simulink library "AnnVolumeBtc"  (R2022b)
settings: Solver=VariableStepAuto  StartTime=0.0  StopTime=10.0  RelTol=1e-3
undefined symbols (not defined in the file or in its folder): Row
libraries: TuneVar x4, TOP x2, FeaturePath x1, HandyTextFile x1, RTC x1, RgainyBtc x1
settings Model: Creator=yp1048186  LastModifiedBy=kl13806
settings SolverCC: AlgebraicLoopSolver=TrustRegion
settings DebuggingCC: UnconnectedInputMsg=warning  UnconnectedOutputMsg=warning  UnconnectedLineMsg=warning  SFMachineParentedDataDiag=warning
settings ModelReferenceCC: EnableRefExpFcnMdlSchedulingChecks=on
settings RTWCC: DLArmComputeVersion=19.05

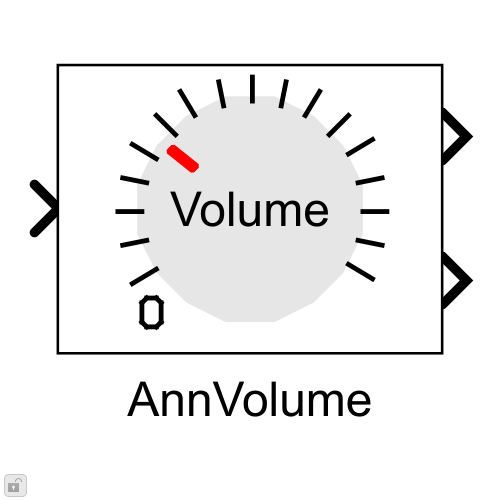
[thumbnail: Simulink's stored preview of the top-level diagram]
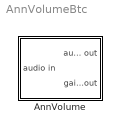
== system AnnVolumeBtc ==
  AnnVolume : Subsystem  mask(Blocklib AnnVolume){FeatureName=Volume, Config=[], TriggerInit=[815 415 895 475]}
      mask prompts: FeatureName "Feature path name:"; Config "AnnVolumeConfig"; TriggerInit "Hidden: MoveFcn redraw"
      mask help: This volume signal block includes receipt of volume level (via RTC) as well as tuning variables to calibrate a gain table that maps 8-bit integer volume index (from RTC) to float decibels.
      mask init:
      | blkh=gcbh;
      | Config=BTConfig.Assert(blkh,Config);
      | BTConfig.InitSetFeatureIfPresent(blkh,'FeatureName');
      | Config.Validate();
      settings: MoveFcn=VolumeMask.CB_TriggerInit(gcbh);
      mask TypeOptions FeatureName: FeaturePath/FeatureName
      mask Callback Config: BTConfig.CallbackHideIfPresent(gcbh,{'FeatureName'});
      mask Callback TriggerInit: VolumeMask.CB_TriggerInit(gcbh);
      mask Display:
      | [path,w,h] = IconVolumeMask();
      | 
      | % work in pixels since the icon does not scale
      | pos = get(gcbh,'position');
      | bw = pos(3) - pos(1);
      | bh = pos(4) - pos(2);
      | 
      | % Draw centered icon
      | xAdj = bw/2 - w/2;
      | yAdj = bh/2 - h/2;
      | for i=1:length(path)
      |     if (path(i).rgb(1) >= 0)
      |         patch(path(i).x+xAdj, path(i).y+yAdj, path(i).rgb);
      |     end
      |     if (path(i).stroke(1) >= 0)
      |         plot(path(i).x+xAdj, path(i).y+yAdj);
      |     end
      | end
      | 
      | % Display some text
      | text(bw/2, bh/2,FeatureName, ...
      |     'horizontalAlignment','center', ...
      |     'VerticalAlignment','middle');

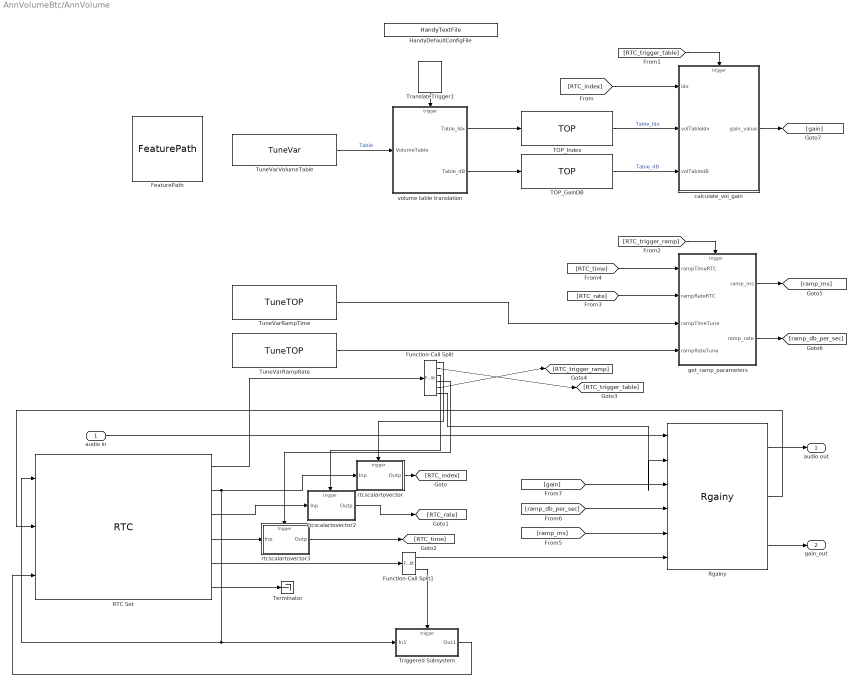
== system AnnVolumeBtc/AnnVolume ==
  audio in : Inport
  FeaturePath : FeaturePath/FeaturePath  FeatureName=Volume  IsGroup=off  GroupNumber=-1  IsModule=off  TriggerInit=[-260 -306 -145 -199]
      settings: SourceProductName=Bose Talaria
  Function-Call Split : FunctionCallSplit  IconShape=distinctive  NumOutputPorts=6
  Function-Call Split1 : FunctionCallSplit  IconShape=distinctive  NumOutputPorts=2  OutputPortLayout=default
  HandyDefaultConfigFile : HandyTextFile/HandyTextFile  TemplateSource=Config  FileSuffix=Init  OpenDialogOnLoad=off  UseThisBlockName=off  TheDefaultText=|  ShowInLibBrowser=on
      | % $(FILENAME) Setup model parameters for each "Init" callback (e.g. update diagram)
      | sample_rate_in_hertz = 44100;
      | frame_size = 32;
      | sysin_channel_count = 2;
      settings: SourceProductName=Bose Talaria
  RTC Set : RTC/RTC  Description=|  REQ_Priority=RTC_Mask.NormalPriority  RequestAtInit=off  EnableRequest=on  REQElemName1=volume_index  REQElemType1=uint32  REQElemWidth1=Config.NumInputChannels  REQElemInitial1=[]  REQElemName2=db_per_second  REQElemType2=uint32  REQElemWidth2=Config.NumInputChannels  REQElemInitial2=[]  REQElemName3=ramp_milliseconds  REQElemType3=uint32  REQElemWidth3=Config.NumInputChannels  REQElemInitial3=[]  REQElemType4=uint32  REQElemWidth4=1  REQElemInitial4=[]  REQElemType5=uint32  REQElemWidth5=1  REQElemInitial5=[]  REQElemType6=uint32  REQElemWidth6=1  REQElemInitial6=[]  REQElemType7=uint32  REQElemWidth7=1  REQElemInitial7=[]  REQElemType8=uint32  REQElemWidth8=1  REQElemInitial8=[]  REQElemType9=uint32  REQElemWidth9=1  REQElemInitial9=[]  REQElemType10=uint32  REQElemWidth10=1  REQElemInitial10=[]  EnableResponse=on  EnableRSP_StatusIn=off  RSPElemName1=gain_index  RSPElemType1=uint32  RSPElemWidth1=Config.NumInputChannels  RSPElemType2=uint32  RSPElemWidth2=1  RSPElemType3=uint32  RSPElemWidth3=1  RSPElemType4=uint32  RSPElemWidth4=1  RSPElemType5=uint32  RSPElemWidth5=1  RSPElemType6=uint32  RSPElemWidth6=1  RSPElemType7=uint32  RSPElemWidth7=1  RSPElemType8=uint32  RSPElemWidth8=1  RSPElemType9=uint32  RSPElemWidth9=1  RSPElemType10=uint32  RSPElemWidth10=1  EnableNotification=on  EnableNTF_PrepTrig=on  NTFElemName1=gain_index  NTFElemType1=uint32  NTFElemWidth1=Config.NumInputChannels  NTFElemType2=uint32  NTFElemWidth2=1  NTFElemType3=uint32  NTFElemWidth3=1  NTFElemType4=uint32  NTFElemWidth4=1  NTFElemType5=uint32  NTFElemWidth5=1  NTFElemType6=uint32  NTFElemWidth6=1  NTFElemType7=uint32  NTFElemWidth7=1  NTFElemType8=uint32  NTFElemWidth8=1  NTFElemType9=uint32  NTFElemWidth9=1  NTFElemType10=uint32  NTFElemWidth10=1  MaskMessageName=Set
      | Sets new target volume.
      | Provide the target volume as 8 bit index value to be mapped through a tunable VolumeTable.
      |  
      | To use slope-based ramping:
      | ----------------------------------
      | When db_per_second has a non-zero value,ramp_milliseconds is ignored and db_per_second controls the ramp.
      |  
      | To use time-based ramping:
      | ----------------------------------
      | The value of db_per_second must be zero for ramp milliseconds to then control the ramping.
      settings: SourceProductName=Bose Talaria
  Rgainy : RgainyBtc/Rgainy  GainOutEnable=on  Config=Config.Rgainy
  TOP_GainDB : TOP/TOP  TriggerInit=[380 -243 530 -187]  TopName=Table_dB  DataType=Inherit: Same as input  BankNumber=Config.BankNumber  PreOverlay=false  PostOverlay=false  Role=Automatic
      settings: SourceProductName=Bose Talaria
  TOP_Index : TOP/TOP  TriggerInit=[380 -313 530 -257]  TopName=Table_Idx  DataType=Inherit: Same as input  BankNumber=Config.BankNumber  PreOverlay=false  PostOverlay=false  Role=Automatic
      settings: SourceProductName=Bose Talaria
  Terminator : Terminator
  TranslateTrigger1 : TuneVar/TranslateTrigger  TriggerInit=[211 -395 249 -345]
      settings: SourceProductName=Bose Talaria
  Triggered Subsystem : Subsystem  TreatAsAtomicUnit=on
  TuneVarRampRate : TuneVar/TuneTOP  TriggerInit=[-95 52 75 108]  TopName=RampRate  TuneName=RampRate  DataType=single  TunabilityNumber=2  MinValue=5  MaxValue=50000  BankNumber=0  PreOverlay=false  PostOverlay=false  UseSameName=on  MaskValue=100
      settings: SourceProductName=Bose Talaria
  TuneVarRampTime : TuneVar/TuneTOP  TriggerInit=[-95 -28 75 28]  TopName=RampTime  TuneName=RampTime  DataType=single  TunabilityNumber=1  MinValue=[]  MaxValue=[]  BankNumber=0  PreOverlay=false  PostOverlay=false  UseSameName=on  MaskValue=100
      settings: SourceProductName=Bose Talaria
  TuneVarVolumeTable : TuneVar/TuneVar  Description=|  TuneName=Table  SpecifyMaxSize=on  VariableDim=1 (Row)  MaxSize=[16 2]  TunabilityNumber=2  MinValue=[0;-100]  MaxValue=[1;0]  TriggerInit=[-95 -275 75 -225]  MaskValue=[[1 32 64 96 128 160 192 224] / 255; [-126.5 -100 -90 -40 -30 -20 -10 0.0]]'
      | <HTML>Gain table maps index to gain.
      | The index values are <FONT color="red">normalized</Font> floats between 0 and 1 while the gains are in dB (i.e. 0 implies no attenuation).
      | </html>
      settings: SourceProductName=Bose Talaria
  calculate_vol_gain : MATLAB Function  TreatAsAtomicUnit=on
  get_ramp_parameters : MATLAB Function  TreatAsAtomicUnit=on
  rtcscalartovector : MATLAB Function  TreatAsAtomicUnit=on
  rtcscalartovector2 : MATLAB Function  TreatAsAtomicUnit=on
  rtcscalartovector3 : MATLAB Function  TreatAsAtomicUnit=on
  volume table translation : MATLAB Function  TreatAsAtomicUnit=on
  audio out : Outport  VectorParamsAs1DForOutWhenUnconnected=off
  gain_out : Outport  Port=2  VectorParamsAs1DForOutWhenUnconnected=off
  wires:
  Rgainy/1 -> audio out/1
  volume table translation/2(Table_dB) -> TOP_GainDB/1
  volume table translation/1(Table_Idx) -> TOP_Index/1
  TuneVarVolumeTable/1 -> volume table translation/1(VolumeTable)  "Table"
  TranslateTrigger1/1 -> volume table translation/Trigger
  TOP_Index/1 -> calculate_vol_gain/2(volTableIdx)  "Table_Idx"
  TOP_GainDB/1 -> calculate_vol_gain/3(volTabledB)  "Table_dB"
  audio in/1 -> Rgainy/1
  RTC Set/1 -> Function-Call Split/1
  Rgainy/2 -> RTC Set/2
  RTC Set/6 -> Terminator/1
  TuneVarRampRate/1 -> get_ramp_parameters/4(rampRateTune)
  TuneVarRampTime/1 -> get_ramp_parameters/3(rampTimeTune)
  RTC Set/3 -> rtcscalartovector2/1(Inp)
  [RTC_index] -> calculate_vol_gain/1(idx)
  [RTC_trigger_table] -> calculate_vol_gain/Trigger
  [RTC_trigger_ramp] -> get_ramp_parameters/Trigger
  [RTC_rate] -> get_ramp_parameters/2(rampRateRTC)
  [RTC_time] -> get_ramp_parameters/1(rampTimeRTC)
  get_ramp_parameters/1(ramp_ms) -> [ramp_ms]
  [ramp_ms] -> Rgainy/5
  get_ramp_parameters/2(ramp_rate) -> [ramp_db_per_sec]
  [ramp_db_per_sec] -> Rgainy/4
  calculate_vol_gain/1(gain_value) -> [gain]
  [gain] -> Rgainy/3
  rtcscalartovector2/1(Outp) -> [RTC_rate]
  rtcscalartovector3/1(Outp) -> [RTC_time]
  RTC Set/2 -> RTC Set/1, Triggered Subsystem/1(In1), rtcscalartovector/1(Inp)
  rtcscalartovector/1(Outp) -> [RTC_index]
  RTC Set/4 -> rtcscalartovector3/1(Inp)
  Rgainy/3 -> gain_out/1
  Function-Call Split/1 -> rtcscalartovector/Trigger
  Function-Call Split/2 -> [RTC_trigger_table]
  Function-Call Split/5 -> [RTC_trigger_ramp]
  Function-Call Split/6 -> Rgainy/2
  Function-Call Split/4 -> rtcscalartovector3/Trigger
  Function-Call Split/3 -> rtcscalartovector2/Trigger
  Triggered Subsystem/1(Out1) -> RTC Set/3
  RTC Set/5 -> Function-Call Split1/1
  Function-Call Split1/1 -> Rgainy/6
  Function-Call Split1/2 -> Triggered Subsystem/Trigger

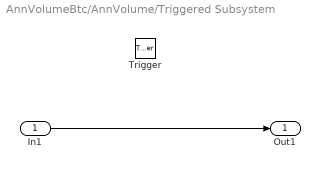
== system AnnVolumeBtc/AnnVolume/Triggered Subsystem ==
  In1 : Inport
  Trigger : TriggerPort  TriggerType=function-call  VariantControl=Variant
  Out1 : Outport
  wires:
  In1/1 -> Out1/1

== matlab function AnnVolumeBtc/AnnVolume/get_ramp_parameters ==
  data: rampTimeRTC input; ramp_ms output; rampRateRTC input; rampTimeTune input; rampRateTune input; ramp_rate output
  events: trigger input FUNCTION_CALL_EVENT
function [ramp_ms, ramp_rate] = get_ramp_parameters(...
    rampTimeRTC, rampRateRTC,... % RTC message parameters
    rampTimeTune, rampRateTune) % Tune parameters

% Ramp time and rate are provided to the block through RTC messages. However 
% in case neither of them are provided, the block will use the default ramp 
% time given in the tune variables.
% NOTE: Tune variable for ramp rate is provided as an option, but not used
% in the current version.
    Numiters=size(rampTimeRTC,2);
    ramp_ms=zeros(1,Numiters);
    ramp_rate=zeros(1,Numiters);

    ramp_ms(1:Numiters) = single(rampTimeTune);
    ramp_rate(1:Numiters) = single(0.0); % Set to rampRateTune if a default is to be set
for rampind=1:Numiters
    if (rampTimeRTC(rampind))
        ramp_ms(rampind) = single(rampTimeRTC(rampind));
        ramp_ms(rampind) = min(100000, ramp_ms(rampind));
        ramp_ms(rampind) = max(1, ramp_ms(rampind));
    end
    if (rampRateRTC(rampind))
        ramp_rate(rampind) = single(rampRateRTC(rampind));
        ramp_rate(rampind) = min(50000, ramp_rate(rampind));
        ramp_rate(rampind) = max(5, ramp_rate(rampind));
    end
end

== matlab function AnnVolumeBtc/AnnVolume/calculate_vol_gain ==
  data: idx input; gain_value output; volTableIdx input; volTabledB input
  events: trigger input FUNCTION_CALL_EVENT
function gain_value = Calculate_Vol_Table(idx, volTableIdx, volTabledB)
%#codegen
% Calculate a gain_value from VolumeTable, table index, and index table
%
iter=size(idx,2);
%gain_value = single(0.0);
gain_value=single(zeros(1,iter));
percent =zeros(1,iter);
lastIdx =zeros(1,iter);

for chind=1:iter
  j = uint8(1);
% workaround to type problem
idx(chind) = cast(idx(chind), class(volTableIdx(end)));

%  bounds checking for vol - clip to max idx
if (idx(chind) > volTableIdx(end))
    idx(chind) = volTableIdx(end);
end

% search through volume table to find index closest to vol
while (j <= numel(volTableIdx))
    if (idx(chind) <= volTableIdx(j))
        if (j <= 1)  % first indexed value is linearly interpolated to zero
            if (volTableIdx(j))
                percent(chind) = single(idx(chind)) / single(volTableIdx(j));
            else
                percent(chind) = single(1);
            end
            gain_value(chind) = percent(chind) * 10 ^ (volTabledB(j) / 20);
        else         % other values are interpolated in db space
            lastIdx(chind) = volTableIdx(j-1);
            percent(chind) = single(idx(chind) - lastIdx(chind)) / single(volTableIdx(j) - lastIdx(chind));
            gain_value(chind) = 10 ^ (((percent(chind) * (volTabledB(j) - volTabledB(j-1))) + volTabledB(j-1)) / 20);
        end
        break;
    else
        j = j + 1;
    end
end
end

== matlab function AnnVolumeBtc/AnnVolume/rtcscalartovector ==
  data: Outp output; Inp input
  events: trigger input FUNCTION_CALL_EVENT
function Outp  = fcn(Inp)
%
% Convert input vector into a matrix
%
%
Inpsize=size(Inp,1);
%#codegen
Outp=(Inp').*uint32(ones(1,Inpsize));

== matlab function AnnVolumeBtc/AnnVolume/volume table translation ==
  data: Table_Idx output; Table_dB output; VolumeTable input
  events: trigger input FUNCTION_CALL_EVENT
function [Table_Idx,Table_dB] = fcn(VolumeTable)
%#codegen
%
% Demux Volume Table matrix into an index vector amd gain vector
%

% Set up the size and datatype of our TOP outputs:
maxTableSize = numel(VolumeTable.Value) / 2;
idxType = 'uint8';
idxStorageType = 'uint32';
dbType = 'single';
Table_Idx = zeros(1,maxTableSize,idxStorageType);
Table_dB = zeros(1,maxTableSize,dbType);

% separate the pairs into their index and value components
givenPairs = VolumeTable.Size(1);
indexes = VolumeTable.Value(1:givenPairs,1);
values = VolumeTable.Value(1:givenPairs,2);

% then sort and ignore duplicates
[cleanIdx,map] = unique(indexes);

% Validate input sizes
numPairs = numel(map);
argName='VolumeTable';

% Validate: enough data?
if (numPairs < 2)
    TranslateError('%s must have at least 2 index pairs. Encounted value with only %f pairs\n', argName, numPairs);
end

% Validate: Highest index still below 1.0?
if (cleanIdx(end) > 1)
    TranslateError('%s out of range table index %f encountered. Index must be between 0 and 1.\n',argName,cleanIdx(end));
end

% fill in the table buffer with provided pairs
for i=1:numPairs
    Table_Idx(i) = intmax(idxType) * cleanIdx(i);
    Table_dB(i) = values(map(i));
end
% fill the rest of the table buffer with the last entry
for j=numel(map)+1:maxTableSize
    Table_Idx(j) = Table_Idx(numPairs);
    Table_dB(j) =  Table_dB(numPairs);
end

end

== matlab function AnnVolumeBtc/AnnVolume/rtcscalartovector2 ==
  data: Outp output; Inp input
  events: trigger input FUNCTION_CALL_EVENT
function Outp  = fcn(Inp)
%
% Convert input vector into a matrix
%
Inpsize=size(Inp,1);
%#codegen
Outp=(Inp').*uint32(ones(1,Inpsize));

== matlab function AnnVolumeBtc/AnnVolume/rtcscalartovector3 ==
  data: Outp output; Inp input
  events: trigger input FUNCTION_CALL_EVENT
function Outp  = fcn(Inp)
%
% Convert input vector into a matrix
%
Inpsize=size(Inp,1);
%#codegen
Outp=(Inp').*uint32(ones(1,Inpsize));
